simulink model "fir_filter_model"  (R2019b)
settings: Solver=FixedStepAuto  StartTime=0.0  StopTime=length(x)-1  RelTol=1e-3
model workspace (MAT data in the model file):
  T.coefficient = embedded.fi
  T.coefficient.DataType = 'Fixed'
  T.coefficient.Scaling = 'BinaryPoint'
  T.coefficient.Signed = 1
  T.coefficient.WordLength = 16
  T.coefficient.FixedExponent = -16
  T.coefficient.SlopeAdjustmentFactor = 1
  T.coefficient.Bias = 0
  T.coefficient.DataTypeOverride = 'Inherit'
  T.coefficient.noverflows = 0
  T.coefficient.nunderflows = 0
  T.coefficient.maxlog = -1.79769313486e+308
  T.coefficient.minlog = 1.79769313486e+308
  T.coefficient.RoundingMethod = 'Floor'
  T.coefficient.OverflowAction = 'Wrap'
  T.coefficient.ProductMode = 'FullPrecision'
  T.coefficient.SumMode = 'SpecifyPrecision'
  T.coefficient.ProductWordLength = 32
  T.coefficient.SumWordLength = 32
  T.coefficient.MaxProductWordLength = 65535
  T.coefficient.MaxSumWordLength = 65535
  T.coefficient.ProductFractionLength = 30
  T.coefficient.ProductFixedExponent = -30
  T.coefficient.ProductSlope = 9.31322574615e-10
  T.coefficient.ProductSlopeAdjustmentFactor = 1
  T.coefficient.ProductBias = 0
  T.coefficient.SumFractionLength = 30
  T.coefficient.SumFixedExponent = -30
  T.coefficient.SumSlope = 9.31322574615e-10
  T.coefficient.SumSlopeAdjustmentFactor = 1
  T.coefficient.SumBias = 0
  T.coefficient.CastBeforeSum = 1
  T.coefficient.DDGMaxProductWordLength = 65535
  T.coefficient.DDGMaxSumWordLength = 65535
  T.coefficient.DDGProductFixedExponent = -30
  T.coefficient.DDGProductFractionLength = 30
  T.coefficient.DDGProductWordLength = 32
  T.coefficient.DDGSumFixedExponent = -30
  T.coefficient.DDGSumFractionLength = 30
  T.coefficient.DDGSumWordLength = 32
  T.coefficient.DDGCastBeforeSum = 1
  T.coefficient.DDGProductBias = 0
  T.coefficient.DDGProductSlopeAdjustmentFactor = 1
  T.coefficient.DDGSumBias = 0
  T.coefficient.DDGSumSlopeAdjustmentFactor = 1
  T.coefficient.DDGProductSlope = 9.31322574615e-10
  T.coefficient.DDGSumSlope = 9.31322574615e-10
  T.coefficient.Logging = 0
  T.coefficient.fimathislocal = 1
  T.input = embedded.fi
  T.input.DataType = 'Fixed'
  T.input.Scaling = 'BinaryPoint'
  T.input.Signed = 1
  T.input.WordLength = 16
  T.input.FixedExponent = -14
  T.input.SlopeAdjustmentFactor = 1
  T.input.Bias = 0
  T.input.DataTypeOverride = 'Inherit'
  T.input.noverflows = 0
  T.input.nunderflows = 0
  T.input.maxlog = -1.79769313486e+308
  T.input.minlog = 1.79769313486e+308
  T.input.RoundingMethod = 'Floor'
  T.input.OverflowAction = 'Wrap'
  T.input.ProductMode = 'FullPrecision'
  T.input.SumMode = 'SpecifyPrecision'
  T.input.ProductWordLength = 32
  T.input.SumWordLength = 32
  T.input.MaxProductWordLength = 65535
  T.input.MaxSumWordLength = 65535
  T.input.ProductFractionLength = 30
  T.input.ProductFixedExponent = -30
  T.input.ProductSlope = 9.31322574615e-10
  T.input.ProductSlopeAdjustmentFactor = 1
  T.input.ProductBias = 0
  T.input.SumFractionLength = 30
  T.input.SumFixedExponent = -30
  T.input.SumSlope = 9.31322574615e-10
  T.input.SumSlopeAdjustmentFactor = 1
  T.input.SumBias = 0
  T.input.CastBeforeSum = 1
  T.input.DDGMaxProductWordLength = 65535
  T.input.DDGMaxSumWordLength = 65535
  T.input.DDGProductFixedExponent = -30
  T.input.DDGProductFractionLength = 30
  T.input.DDGProductWordLength = 32
  T.input.DDGSumFixedExponent = -30
  T.input.DDGSumFractionLength = 30
  T.input.DDGSumWordLength = 32
  T.input.DDGCastBeforeSum = 1
  T.input.DDGProductBias = 0
  T.input.DDGProductSlopeAdjustmentFactor = 1
  T.input.DDGSumBias = 0
  T.input.DDGSumSlopeAdjustmentFactor = 1
  T.input.DDGProductSlope = 9.31322574615e-10
  T.input.DDGSumSlope = 9.31322574615e-10
  T.input.Logging = 0
  T.input.fimathislocal = 1
  T.output = embedded.fi
  T.output.DataType = 'Fixed'
  T.output.Scaling = 'BinaryPoint'
  T.output.Signed = 1
  T.output.WordLength = 16
  T.output.FixedExponent = -14
  T.output.SlopeAdjustmentFactor = 1
  T.output.Bias = 0
  T.output.DataTypeOverride = 'Inherit'
  T.output.noverflows = 0
  T.output.nunderflows = 0
  T.output.maxlog = -1.79769313486e+308
  T.output.minlog = 1.79769313486e+308
  T.output.RoundingMethod = 'Floor'
  T.output.OverflowAction = 'Wrap'
  T.output.ProductMode = 'FullPrecision'
  T.output.SumMode = 'SpecifyPrecision'
  T.output.ProductWordLength = 32
  T.output.SumWordLength = 32
  T.output.MaxProductWordLength = 65535
  T.output.MaxSumWordLength = 65535
  T.output.ProductFractionLength = 30
  T.output.ProductFixedExponent = -30
  T.output.ProductSlope = 9.31322574615e-10
  T.output.ProductSlopeAdjustmentFactor = 1
  T.output.ProductBias = 0
  T.output.SumFractionLength = 30
  T.output.SumFixedExponent = -30
  T.output.SumSlope = 9.31322574615e-10
  T.output.SumSlopeAdjustmentFactor = 1
  T.output.SumBias = 0
  T.output.CastBeforeSum = 1
  T.output.DDGMaxProductWordLength = 65535
  T.output.DDGMaxSumWordLength = 65535
  T.output.DDGProductFixedExponent = -30
  T.output.DDGProductFractionLength = 30
  T.output.DDGProductWordLength = 32
  T.output.DDGSumFixedExponent = -30
  T.output.DDGSumFractionLength = 30
  T.output.DDGSumWordLength = 32
  T.output.DDGCastBeforeSum = 1
  T.output.DDGProductBias = 0
  T.output.DDGProductSlopeAdjustmentFactor = 1
  T.output.DDGSumBias = 0
  T.output.DDGSumSlopeAdjustmentFactor = 1
  T.output.DDGProductSlope = 9.31322574615e-10
  T.output.DDGSumSlope = 9.31322574615e-10
  T.output.Logging = 0
  T.output.fimathislocal = 1
  T.sum = embedded.fi
  T.sum.DataType = 'Fixed'
  T.sum.Scaling = 'BinaryPoint'
  T.sum.Signed = 1
  T.sum.WordLength = 32
  T.sum.FixedExponent = -30
  T.sum.SlopeAdjustmentFactor = 1
  T.sum.Bias = 0
  T.sum.DataTypeOverride = 'Inherit'
  T.sum.noverflows = 0
  T.sum.nunderflows = 0
  T.sum.maxlog = -1.79769313486e+308
  T.sum.minlog = 1.79769313486e+308
  T.sum.RoundingMethod = 'Floor'
  T.sum.OverflowAction = 'Wrap'
  T.sum.ProductMode = 'FullPrecision'
  T.sum.SumMode = 'SpecifyPrecision'
  T.sum.ProductWordLength = 32
  T.sum.SumWordLength = 32
  T.sum.MaxProductWordLength = 65535
  T.sum.MaxSumWordLength = 65535
  T.sum.ProductFractionLength = 30
  T.sum.ProductFixedExponent = -30
  T.sum.ProductSlope = 9.31322574615e-10
  T.sum.ProductSlopeAdjustmentFactor = 1
  T.sum.ProductBias = 0
  T.sum.SumFractionLength = 30
  T.sum.SumFixedExponent = -30
  T.sum.SumSlope = 9.31322574615e-10
  T.sum.SumSlopeAdjustmentFactor = 1
  T.sum.SumBias = 0
  T.sum.CastBeforeSum = 1
  T.sum.DDGMaxProductWordLength = 65535
  T.sum.DDGMaxSumWordLength = 65535
  T.sum.DDGProductFixedExponent = -30
  T.sum.DDGProductFractionLength = 30
  T.sum.DDGProductWordLength = 32
  T.sum.DDGSumFixedExponent = -30
  T.sum.DDGSumFractionLength = 30
  T.sum.DDGSumWordLength = 32
  T.sum.DDGCastBeforeSum = 1
  T.sum.DDGProductBias = 0
  T.sum.DDGProductSlopeAdjustmentFactor = 1
  T.sum.DDGSumBias = 0
  T.sum.DDGSumSlopeAdjustmentFactor = 1
  T.sum.DDGProductSlope = 9.31322574615e-10
  T.sum.DDGSumSlope = 9.31322574615e-10
  T.sum.Logging = 0
  T.sum.fimathislocal = 1
  T.index = []
  b = embedded.fi
  b.DataType = 'Fixed'
  b.Scaling = 'BinaryPoint'
  b.Signed = 1
  b.WordLength = 16
  b.FixedExponent = -16
  b.SlopeAdjustmentFactor = 1
  b.Bias = 0
  b.DataTypeOverride = 'Inherit'
  b.intarray = [-42 -120 -168 -105 155 546 773 442 -602 -1949 -2610 -1462 2033 7283 12612 15973 15973 12612 7283 2033 -1462 -2610 -1949 -602 442 773 546 155 -105 -168 -120 -42]
  b.noverflows = 0
  b.nunderflows = 0
  b.maxlog = -1.79769313486e+308
  b.minlog = 1.79769313486e+308
  b.RoundingMethod = 'Floor'
  b.OverflowAction = 'Wrap'
  b.ProductMode = 'FullPrecision'
  b.SumMode = 'SpecifyPrecision'
  b.ProductWordLength = 32
  b.SumWordLength = 32
  b.MaxProductWordLength = 65535
  b.MaxSumWordLength = 65535
  b.ProductFractionLength = 30
  b.ProductFixedExponent = -30
  b.ProductSlope = 9.31322574615e-10
  b.ProductSlopeAdjustmentFactor = 1
  b.ProductBias = 0
  b.SumFractionLength = 30
  b.SumFixedExponent = -30
  b.SumSlope = 9.31322574615e-10
  b.SumSlopeAdjustmentFactor = 1
  b.SumBias = 0
  b.CastBeforeSum = 1
  b.DDGMaxProductWordLength = 65535
  b.DDGMaxSumWordLength = 65535
  b.DDGProductFixedExponent = -30
  b.DDGProductFractionLength = 30
  b.DDGProductWordLength = 32
  b.DDGSumFixedExponent = -30
  b.DDGSumFractionLength = 30
  b.DDGSumWordLength = 32
  b.DDGCastBeforeSum = 1
  b.DDGProductBias = 0
  b.DDGProductSlopeAdjustmentFactor = 1
  b.DDGSumBias = 0
  b.DDGSumSlopeAdjustmentFactor = 1
  b.DDGProductSlope = 9.31322574615e-10
  b.DDGSumSlope = 9.31322574615e-10
  b.Logging = 0
  b.fimathislocal = 1
  x = embedded.fi
  x.DataType = 'Fixed'
  x.Scaling = 'BinaryPoint'
  x.Signed = 1
  x.WordLength = 16
  x.FixedExponent = -14
  x.SlopeAdjustmentFactor = 1
  x.Bias = 0
  x.DataTypeOverride = 'Inherit'
  x.intarray = [0 51 205 463 823 1285 1849 2512 3272 4124 5062 6079 ... (411 elements, 411x1)]
  x.noverflows = 0
  x.nunderflows = 0
  x.maxlog = -1.79769313486e+308
  x.minlog = 1.79769313486e+308
  x.RoundingMethod = 'Floor'
  x.OverflowAction = 'Wrap'
  x.ProductMode = 'FullPrecision'
  x.SumMode = 'SpecifyPrecision'
  x.ProductWordLength = 32
  x.SumWordLength = 32
  x.MaxProductWordLength = 65535
  x.MaxSumWordLength = 65535
  x.ProductFractionLength = 30
  x.ProductFixedExponent = -30
  x.ProductSlope = 9.31322574615e-10
  x.ProductSlopeAdjustmentFactor = 1
  x.ProductBias = 0
  x.SumFractionLength = 30
  x.SumFixedExponent = -30
  x.SumSlope = 9.31322574615e-10
  x.SumSlopeAdjustmentFactor = 1
  x.SumBias = 0
  x.CastBeforeSum = 1
  x.DDGMaxProductWordLength = 65535
  x.DDGMaxSumWordLength = 65535
  x.DDGProductFixedExponent = -30
  x.DDGProductFractionLength = 30
  x.DDGProductWordLength = 32
  x.DDGSumFixedExponent = -30
  x.DDGSumFractionLength = 30
  x.DDGSumWordLength = 32
  x.DDGCastBeforeSum = 1
  x.DDGProductBias = 0
  x.DDGProductSlopeAdjustmentFactor = 1
  x.DDGSumBias = 0
  x.DDGSumSlopeAdjustmentFactor = 1
  x.DDGProductSlope = 9.31322574615e-10
  x.DDGSumSlope = 9.31322574615e-10
  x.Logging = 0
  x.fimathislocal = 1
values from neighbouring files (symbols this model uses):
  b = cast(b,'like',T.coefficient)    [test_fir_filter.m]    (also in test_matlab_function_block.m = cast(b0,'like',T.coefficient))
  T = fir_filter_dsp_types    [test_fir_filter.m]    (also in test_matlab_function_block.m)
libraries: dspsrcs4 x1
settings Model: Creator=tbryan  LastModifiedBy=tbryan
settings HardwareCC: ProdBitPerLong=64  ProdHWDeviceType=Intel->x86-64 (Mac OS X)
settings SFSimCC: SimParseCustomCode=off

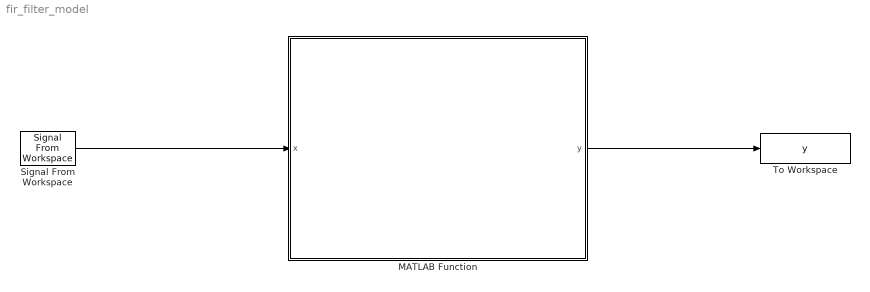
== system fir_filter_model ==
  MATLAB Function : MATLAB Function  TreatAsAtomicUnit=on
  Signal From Workspace : dspsrcs4/Signal From Workspace  X=x  Ts=1  nsamps=1  OutputAfterFinalValue=Setting to zero  ignoreOrWarnInputAndFrameLengths=off  OutputFrames=off
  To Workspace : ToWorkspace  VariableName=y  SampleTime=-1
  wires:
  Signal From Workspace/1 -> MATLAB Function/1(x)
  MATLAB Function/1(y) -> To Workspace/1

== matlab function fir_filter_model/MATLAB Function ==
  data: x input; y output; b parameter; T parameter
function y = fir_filter_matlab_function_block(x,b,T)
    persistent z
    persistent p
    if isempty(z)
        z = zeros(size(b),'like',T.input);
        p = cast(0,'like',T.index);
    end
    [y,z,p] = fir_filter(b,x,z,p,T);
end
